simulink model "CONT_PD_BALANCEO"  (R2024b)
settings: Solver=VariableStepAuto  StartTime=0.0  StopTime=10.0  RelTol=1e-3
undefined symbols (not defined in the file): bt, g, Mt
libraries: simulink x1
settings Model: Creator=juani  LastModifiedBy=juani

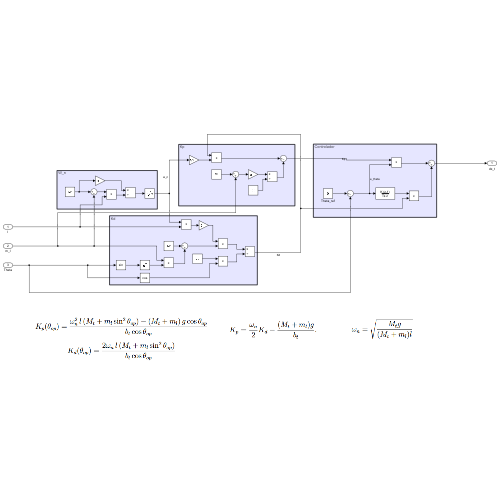
[thumbnail: Simulink's stored preview of the top-level diagram]
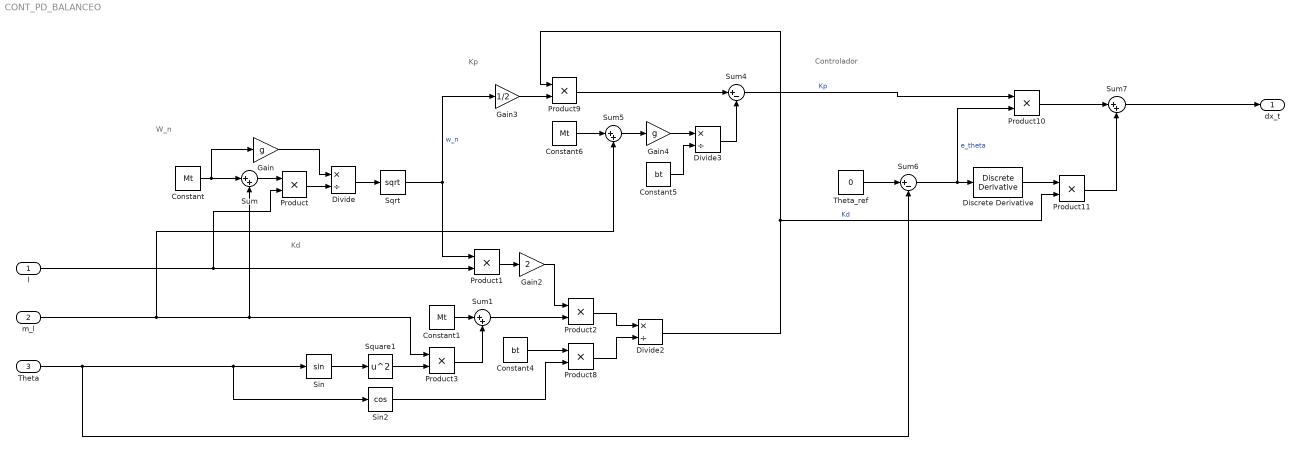
== system CONT_PD_BALANCEO ==
  note: Controlador
  note: Kp
  note: Kd
  note: W_n
  l : Inport
  m_l : Inport  Port=2
  Theta : Inport  Port=3
  Constant : Constant  Value=Mt
  Constant1 : Constant  Value=Mt
  Constant4 : Constant  Value=bt
  Constant5 : Constant  Value=bt
  Constant6 : Constant  Value=Mt
  Discrete Derivative : simulink/Discrete/Discrete Derivative  gainval=1.0  ICPrevScaledInput=0.0  OutMin=[]  OutMax=[]  OutDataType=fixdt(1, 16)  OutScaling=2^-10  DoSatur=off
  Divide : Product  Inputs=*/
  Divide2 : Product  Inputs=*/
  Divide3 : Product  Inputs=*/
  Gain : Gain  Gain=g
  Gain2 : Gain  Gain=2
  Gain3 : Gain  Gain=1/2
  Gain4 : Gain  Gain=g
  Product{,1..3,8..11} (8 alike) : Product
  Sin : Trigonometry
  Sin2 : Trigonometry  Operator=cos
  Sqrt : Sqrt
  Square1 : Math  Operator=square
  Sum{,1,5,7} (4 alike) : Sum  Inputs=|++
  Sum4 : Sum  Inputs=|+-
  Sum6 : Sum  Inputs=|+-
  Theta_ref : Constant  Value=0
  dx_t : Outport
  wires:
  Constant/1 -> Gain/1, Sum/1
  m_l/1 -> Sum/2, Product3/1, Sum5/2
  Sum/1 -> Product/1
  l/1 -> Product/2, Product1/2
  Gain/1 -> Divide/1
  Product/1 -> Divide/2
  Divide/1 -> Sqrt/1
  Sqrt/1 -> Product1/1, Gain3/1  "w_n"
  Constant1/1 -> Sum1/1
  Sin/1 -> Square1/1
  Theta/1 -> Sum6/2, Sin2/1, Sin/1
  Square1/1 -> Product3/2
  Product3/1 -> Sum1/2
  Product1/1 -> Gain2/1
  Gain2/1 -> Product2/1
  Sum1/1 -> Product2/2
  Constant4/1 -> Product8/1
  Sin2/1 -> Product8/2
  Product2/1 -> Divide2/1
  Product8/1 -> Divide2/2
  Divide2/1 -> Product11/2, Product9/1  "Kd"
  Gain3/1 -> Product9/2
  Product9/1 -> Sum4/1
  Constant6/1 -> Sum5/1
  Sum5/1 -> Gain4/1
  Gain4/1 -> Divide3/1
  Constant5/1 -> Divide3/2
  Divide3/1 -> Sum4/2
  Sum4/1 -> Product10/1  "Kp"
  Theta_ref/1 -> Sum6/1
  Sum6/1 -> Product10/2, Discrete Derivative/1  "e_theta"
  Product10/1 -> Sum7/1
  Sum7/1 -> dx_t/1
  Discrete Derivative/1 -> Product11/1
  Product11/1 -> Sum7/2
